simulink model "pmsm_model"  (R2024a)
settings: Solver=VariableStepAuto  StartTime=0.0  StopTime=10.0  RelTol=1e-3
settings Model: Creator=s14  LastModifiedBy=s14

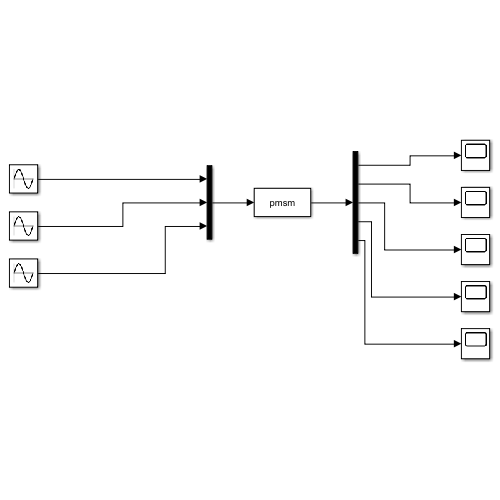
[thumbnail: Simulink's stored preview of the top-level diagram]
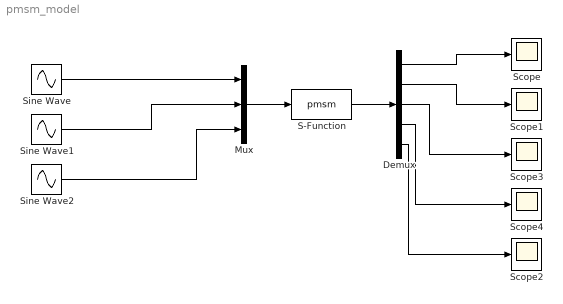
== system pmsm_model ==
  Demux : Demux  Outputs=5
  Mux : Mux  Inputs=3
  S-Function : S-Function  FunctionName=pmsm  SFunctionDeploymentMode=off  EnableBusSupport=off
  Scope{,1..4} (5 alike) : Scope
  Sine Wave : Sin  Amplitude=311  Frequency=2*pi*50  SampleTime=0
  Sine Wave1 : Sin  Amplitude=311  Frequency=2*pi*50  Phase=-2*pi/3  SampleTime=0
  Sine Wave2 : Sin  Amplitude=311  Frequency=2*pi*50  Phase=2*pi/3  SampleTime=0
  wires:
  Mux/1 -> S-Function/1
  S-Function/1 -> Demux/1
  Sine Wave/1 -> Mux/1
  Sine Wave1/1 -> Mux/2
  Sine Wave2/1 -> Mux/3
  Demux/1 -> Scope/1
  Demux/2 -> Scope1/1
  Demux/5 -> Scope2/1
  Demux/3 -> Scope3/1
  Demux/4 -> Scope4/1
